simulink model "laba2"  (R2022a)
settings: Solver=VariableStepAuto  StartTime=0.0  StopTime=10.0  RelTol=1e-3
settings Model: Creator=User  LastModifiedBy=User

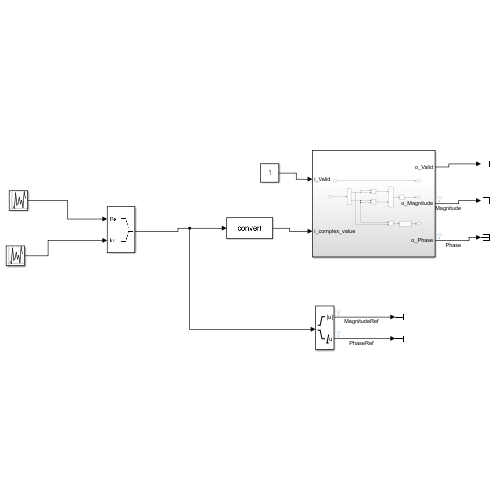
[thumbnail: Simulink's stored preview of the top-level diagram]
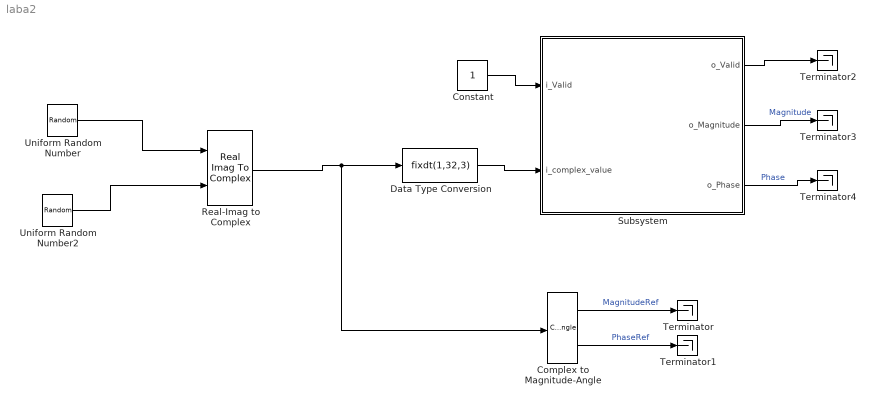
== system laba2 ==
  Complex to Magnitude-Angle : ComplexToMagnitudeAngle
  Constant : Constant  OutDataTypeStr=boolean
  Data Type Conversion : DataTypeConversion  OutDataTypeStr=fixdt(1,32,3)  RndMeth=Round  SaturateOnIntegerOverflow=off
  Real-Imag to Complex : RealImagToComplex
  Subsystem : Subsystem
  Terminator{,1..4} (5 alike) : Terminator
  Uniform Random Number : UniformRandomNumber  Minimum=-2^(29-1)  Maximum=2^(29-1)-1/2^3  Seed=29  SampleTime=1
  Uniform Random Number2 : UniformRandomNumber  Minimum=-2^(29-1)  Maximum=2^(29-1)-1/2^3  Seed=30  SampleTime=1
  wires:
  Uniform Random Number/1 -> Real-Imag to Complex/1
  Uniform Random Number2/1 -> Real-Imag to Complex/2
  Real-Imag to Complex/1 -> Complex to Magnitude-Angle/1, Data Type Conversion/1
  Complex to Magnitude-Angle/1 -> Terminator/1  "MagnitudeRef"
  Complex to Magnitude-Angle/2 -> Terminator1/1  "PhaseRef"
  Constant/1 -> Subsystem/1(i_Valid)
  Data Type Conversion/1 -> Subsystem/2(i_complex_value)
  Subsystem/3(o_Phase) -> Terminator4/1  "Phase"
  Subsystem/2(o_Magnitude) -> Terminator3/1  "Magnitude"
  Subsystem/1(o_Valid) -> Terminator2/1

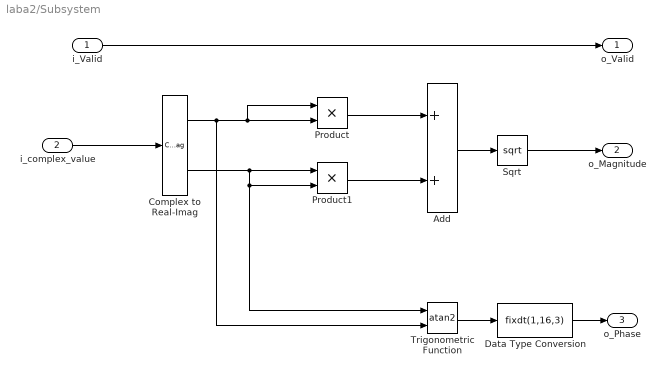
== system laba2/Subsystem ==
  i_Valid : Inport
  i_complex_value : Inport  Port=2
  Add : Sum
  Complex to Real-Imag : ComplexToRealImag
  Data Type Conversion : DataTypeConversion  OutDataTypeStr=fixdt(1,16,3)  RndMeth=Round  SaturateOnIntegerOverflow=off
  Product : Product
  Product1 : Product
  Sqrt : Sqrt  OutDataTypeStr=fixdt(1,33,3)
  Trigonometric Function : Trigonometry  Operator=atan2  ApproximationMethod=CORDIC
  o_Valid : Outport
  o_Magnitude : Outport  Port=2
  o_Phase : Outport  Port=3
  wires:
  Complex to Real-Imag/2 -> Trigonometric Function/1, Product1/2, Product1/1
  i_complex_value/1 -> Complex to Real-Imag/1
  Sqrt/1 -> o_Magnitude/1
  Complex to Real-Imag/1 -> Trigonometric Function/2, Product/2, Product/1
  Product1/1 -> Add/2
  Add/1 -> Sqrt/1
  i_Valid/1 -> o_Valid/1
  Product/1 -> Add/1
  Trigonometric Function/1 -> Data Type Conversion/1
  Data Type Conversion/1 -> o_Phase/1
